simulink model "BuckyWagon_01"  (Simulink 7.7)
settings: Solver=FixedStepDiscrete  StartTime=0.0  StopTime=10.0  RelTol=1e-3
PreLoadFcn:
  | try, eval([bdroot '_setup']); catch, eval('model_setup', ''); end
InitFcn:
  | try, eval([bdroot '_setup']); catch, eval('model_setup', ''); end
undefined symbols (not defined in the file or in its folder): ECU565, High, Low, miniviewSetup, motohawk_build_version, motohawk_get_faults, motohawk_setup_toolchains, motohawk_trunc_name, motohawk_vardec_config_group, motohawk_vardec_path, tc, True
libraries: MotoHawk_lib x594, simulink x27, motohawk_control_primitives_lib x19, miniview_lib x10, MotoHawk_VDOGauge_lib x8, motohawk_engine_lib x5, motohawk_annotations_lib x1
(part 1 of 10)
Description:
  | ESled_08
CloseFcn:
  | try, eval([bdroot '_close']); catch, eval('model_close', ''); end
settings Model: MotoHawkBuildVersion=172  MotoHawkBuildStats=struct('TotalFLASH',{281540},'TotalEEPROM',{370},'TotalRAM',{18696},'AppFLASH',{71914},'AppEEPROM',{196},'AppRAM',{2166},'HeapRAM',{4096},'BuildSuccessCount',{175},'BuildErrorCount',{29},'OSRAM',{4754},'StackRAM',{7680},'FgndTimeStackSize',{3072},'FgndAngleStackSize',{0},'BgndStackSize',{2048},'IdleStackSize',{1024},'InterruptStackSize',{1536},'RTWBlockIOSize',{852},'RTWDWorkSize',{364},'RTWPrevZCSize',{0},'VolatileSize',{272},'NonVolatileSize',{196},'ConstantSize',{2208})  MotoHawkModelSavedName=BuckyWagon_01  MotoHawkModelGUID=3c32a120-d49a-4164-87-fe-ac-4b-55-ed-6f  MotoHawkModelOpenTime=2018 4 23 14 14 23.09  MotoHawkModelElapsedTime=-4921462.717  MotoHawkBuildInfo=struct('model_name',{'BuckyWagon_01'},'motohawk_version',{'2011a_sp0.184'},'motohawk_component_version',{'0.0.7'},'matlab_version',{'7.12.0'},'build_version',{'171'},'module_type',{'ECU565-128'},'layout_type',{'DEV'},'processor_family',{'PPC'},'processor_type',{'MPC565'},'toolchain_vendor',{'gcc-powerpc-eabi'},'toolchain_version',{'4.4.0'},'component',{0},'archive_file',{'PCM128.a'},'enable_build',{1},'fptype',{0},'flash_size',{1048576},'ee_size',{8192},'ram_size',{36864},'decram_size',{4096},'module_memory_def',{'MPC565_ModMemoryDef_Dev'},'eri_table0_rev',{9},'max_eri_table_size',{65535},'use_debug_vardecs',{1},'use_info_vardecs',{1},'fgnd_base_period_ms',{5},'bgnd_base_period_ms',{50},'root_build_dir',{'C:\Users\HYBRID\Documents\GitHub\Wisconsin-Hybrid\BuckyWagon_01'},'build_dir',{'C:\Users\HYBRID\Documents\GitHub\Wisconsin-Hybrid\BuckyWagon_01\BuckyWagon_01_Build'},'dll_name',{'BuckyWago_171'},'srz_name',{'BuckyWagon_01_171'},'fgnd_stack_size',{3072},'fgnd_angle_stack_size',{0},'bgnd_stack_size',{2048},'idle_stack_size',{1024},'irq_stack_size',{1536},'heap_size',{4096},'heap_margin',{409},'install_dll_dir',{'C:\ECUFiles\TDBDLL\'},'install_srz_dir',{'C:\ECUFiles\Programs'},'app_int_stack_size',{1024},'shutdown_stack_size',{1024},'mingw_dir',{'C:\PROGRA~2\Woodward\DEVELO~1\TOOLCH~1\GCC\win32-pe\4_4_0\'},'motohawk_dir',{'C:\PROGRA~2\Woodward\MCS\MotoHawk\2011A_~1.184'},'toolchain_dir',{'C:\Program Files (x86)\Woodward\DevelopmentTools\Toolchains\GCC\powerpc-eabi\4_4_0\'},'matlab_root',{'C:\Program Files (x86)\MATLAB\R2011a'},'model_guid',{'3c32a120-d49a-4164-87-fe-ac-4b-55-ed-6f'},'build_guid',{'f6bced0b-f3ce-4c1d-a0-1c-47-b3-99-ef-d3'},'token_guid',{'DD8AD11F95A6FC42BFF9AC780840E4B4'})  MotoHawkBuildGUID=f6bced0b-f3ce-4c1d-a0-1c-47-b3-99-ef-d3  Creator=Danny  LastModifiedBy=HYBRID
settings OptimizationCC: InlineParams=on  InitFltsAndDblsToZero=on  OptimizeModelRefInitCode=on  LifeSpan=1
settings DebuggingCC: SolverPrmCheckMsg=none  InheritedTsInSrcMsg=none  TasksWithSamePriorityMsg=none  StrictBusMsg=Warning
settings HardwareCC: ProdEndianess=BigEndian  ProdHWDeviceType=Specified
settings SFSimCC: SimCustomHeaderCode=|
  | #include <string.h>
  | #define charPtr(p) ((char *)p)
settings RTWCC: SystemTargetFile=motohawk_ert_rtw.tlc  TLCOptions="-aCustomNonFinites=\"motohawk_genrtnonfinite.tlc\""  MakeCommand=motohawk_make_rtw  TemplateMakefile=motohawk_ert_rtw.tmf  Description=MotoHawk(tm) Rapid Prototyping  ProcessScript=motohawk_ert_rtw_make_rtw_hook
settings CodeAppCC: IgnoreCustomStorageClasses=off  MaxIdLength=100  CustomSymbolStrField=$H$N$M
settings STFCustomTargetCC: FunctionExecutionProfile=off  ModelReferenceCompliant=off  CombineOutputUpdateFcns=on  ERTCustomFileBanners=on  SupportContinuousTime=off  SupportNonInlinedSFcns=off  SystemTargetFile=motohawk_ert_rtw.tlc
settings ERTTargetCC: FunctionExecutionProfile=off  MultiwordLength=2048  ModelReferenceCompliant=off  ParMdlRefBuildCompliant=off  CompOptLevelCompliant=off  ERTFirstTimeCompliant=off  ModelStepFunctionPrototypeControlCompliant=off  CPPClassGenCompliant=off  ERTCustomFileTemplate=example_file_process.tlc  ConvertIfToSwitch=off

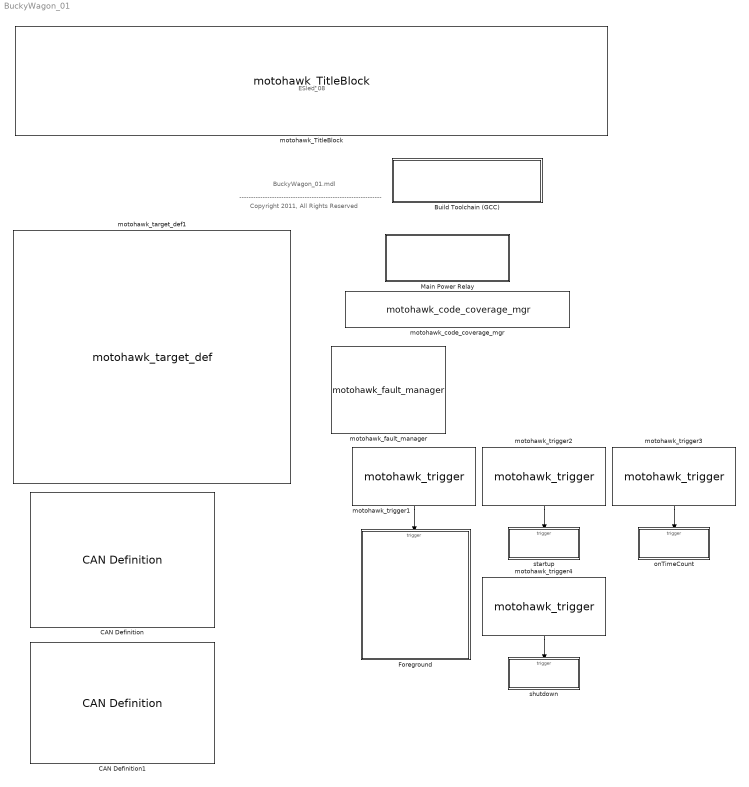
== system BuckyWagon_01 ==
  note: ESled_08
  note: BuckyWagon_01.mdl
  note: -------------------------------------------------------------
  note: Copyright 2011, All Rights Reserved
  Build Toolchain (GCC) : Subsystem
      mask Display:
      | patch([0 0 1 1], [0 1 1 0], [220/255 220/255 220/255]);
      | patch([0 0 1 1], [0 0.075 0.075 0], [230/255 0/255 0/255]);
      | patch([0 0 1 1], [0.025 0.05 0.05 0.025], [150/255 0/255 0/255]);
      | patch([0 0 1 1], [0 0.025 0.025 0], [0/255 0/255 0/255]);
      | 
      | disp(['Build'])
  CAN Definition : MotoHawk_lib/CAN Blocks/CAN Definition  Priority=-100  nam=['CAN_' num2str(1)]  text_resource=CAN1  code_resource=NONE  val_resource=-1  target=ECU565-128  bus=-2  btime=250 kbaud  pre=1  prop=0  pseg1=0  pseg2=0  resyn=0  tx_queue_size=16  rx_queue_size=16  use_protocol=on  city_id=hex2dec('B')  access_level=4  mototune_group='System | System Config | Communication Config'
  CAN Definition1 : MotoHawk_lib/CAN Blocks/CAN Definition  Priority=-100  nam=['CAN_' num2str(2)]  text_resource=CAN2  code_resource=NONE  val_resource=-1  target=ECU565-128  bus=-2  btime=500 kbaud  pre=1  prop=0  pseg1=0  pseg2=0  resyn=0  tx_queue_size=16  rx_queue_size=16  use_protocol=off  city_id=hex2dec('B')  access_level=4  mototune_group='System | System Config | Communication Config'
  Foreground : Subsystem  TreatAsAtomicUnit=on
      settings: RTWSystemCode=Function  RTWFcnNameOpts=Use subsystem name  RTWFileNameOpts=Use function name
  Main Power Relay : Subsystem  AncestorBlock=MotoHawk_lib/Extra Development Blocks/Main Power Relay  mask(MotoHawk Main Power Relay Control){on_delay_count=2, off_delay_count=10, ecup_threshold=100, group='System | Main Power Relay'}
      mask prompts: on_delay_count "On Delay Count"; off_delay_count "Off Delay Count"; ecup_threshold "ECUP High Threshold (ADC Counts)"; group "MotoTune Group"
      mask help:
      | This block provides basic control of the main power relay, by following the ECUP voltage input pin.
      |
      | Regardless of where the block is placed in a design, the strategy will execute every 50ms with background priority.
      |
      | Note that this block is simply composed of other primitive MotoHawk blocks and may be used as a starting point for a more complicated strategy.
      |
      | On Delay:  Once the ECU power goes high, after this period, the Main Power Relay will be turned on.
      | Off Delay:  Once the ECU power goes low, after this period, the Main Power Relay will be turned off.
      |
      | Note that one tick before MPRD is turned off, non-volatile variables will be stored, and the Shutdown event will be posted.  It is not necessary to use the Shutdown event.
      |
      | ---------------------------------------------------------------------
      |
      |
      | Copyright 2010 Woodward.  All Rights Reserved.
      mask init:
      | block = gcb;
      | 
      | motohawk_main_power_relay_initmask;
      mask Help: eval('motohawk_block_help(get_param(gcb,''MaskType''))');
      mask Display:
      | patch([0 0 1 1], [0 1 1 0], [220/255 220/255 220/255]);
      | patch([0 0 1 1], [0 0.075 0.075 0], [230/255 0/255 0/255]);
      | patch([0 0 1 1], [0.025 0.05 0.05 0.025], [150/255 0/255 0/255]);
      | patch([0 0 1 1], [0 0.025 0.025 0], [0/255 0/255 0/255]);
      | 
      | disp(['Main Power Relay' on_delay_lbl off_delay_lbl]);
  motohawk_TitleBlock : motohawk_annotations_lib/motohawk_TitleBlock  BlockType_='Mototron_Title_Block'  ttl="[  strrep(get_param(bdroot, 'Description') , '_', '\\_')  '\\newline\\rm'  'Top-level root of model:  '   strrep(bdroot, '_', '\\_') '.mdl'  ]"  copyright="'THE INFORMATION CONTAINED IN THIS\\newlineDRAWING IS THE SOLE PROPERTY OF\\newlineMOTOTRON.  ANY REPRODUCTION IN\\newline PART OR AS A WHOLE WITHOUT THE\\newlineWRITTEN PERMISSION OF MOTOTRON\\newline IS PROHIBITED.\\fontsize{16}\\rm\\copyright\\rm\\fontsize{10} 2005'"  address='\fontsize{22}\it\fontname{Arial Black}MotoTron Corporation \fontname{Arial}\fontsize{10}\newline505 Marion Road, Oshkosh, WI, 54901\newlinewww.mototron.com (734) 822-7700'  image_file='mh.jpg'  pretty_print=on  edit_text=|  edit_as=5
      | [	
      | 
      | 
      | 	
      | 
      | 
      | strrep(get_param(bdroot, 'Description') , '_', '\_')  '\newline\rm'	
      | 
      | 
      | 	
      | 
      | 
      | 'Top-level root of model:  '   strrep(bdroot, '_', '\_') '.mdl'	
      | 
      | 
      | 	
      | 
      | 
      | ]
  motohawk_code_coverage_mgr : MotoHawk_lib/Extra Development Blocks/motohawk_code_coverage_mgr  codegen=Always Generate Code Coverage Code  group='System | Code Coverage'
  motohawk_fault_manager : MotoHawk_lib/Fault Management Blocks/motohawk_fault_manager  storage=FLASH  read_level=1  write_level=1  clear_level=1  xytype=uint16  mototune_group='Faults'
  motohawk_target_def1 : MotoHawk_lib/motohawk_target_def  Priority=-65535  target=ECU565-128  layout=DEV  fptype=single (32 bits)  fgnd_stack_size=3*1024  fgnd_angle_stack_size=0  bgnd_stack_size=2*1024  idle_stack_size=1024  irq_stack_size=1536  app_int_stack_size=1024  shutdown_stack_size=1024  heap_size=4*1024  show_margins=off  fgnd_stack_margin=(3*1024) * 0.1  fgnd_angle_stack_margin=0  bgnd_stack_margin=(2*1024) * 0.1  idle_stack_margin=(1024) * 0.1  irq_stack_margin=(1536) * 0.1  app_int_stack_margin=(1024) * 0.1  shutdown_stack_margin=(1024) * 0.1  heap_margin=(4*1024) * 0.1  comp_name=bdroot  comp_img='KVASER_CAN_USB.jpg'  comp_security=No Encryption  comp_build_pass='mhbuild'  comp_sim_pass='mhsim'  comp_multi=off  show_filenames=off  dll_name=motohawk_trunc_name(bdroot, ['_' motohawk_build_version], 13)  srz_name=motohawk_trunc_name(bdroot, ['_' motohawk_build_version], 50)  build_dir='.'  comp_dir='.'
  motohawk_trigger1 : MotoHawk_lib/Trigger Blocks/motohawk_trigger  Tag=Trigger  trigger=FGND_RTI_PERIODIC  function_name=Trigger_FGND_RTI_PERIODIC_4287p0005  priority_order=0  inherited=off  run_disabled=off  override_app_monitor=off  target=ECU565_128
  motohawk_trigger2 : MotoHawk_lib/Trigger Blocks/motohawk_trigger  Tag=Trigger  trigger=STARTUP_EVENT  function_name=Trigger_STARTUP_EVENT_4288p0005  priority_order=0  inherited=off  run_disabled=off  override_app_monitor=off  target=ECU565_128
  motohawk_trigger3 : MotoHawk_lib/Trigger Blocks/motohawk_trigger  Tag=Trigger  trigger=BGND_BASEx20_PERIODIC  function_name=Trigger_BGND_BASEx20_PERIODIC_4289p0005  priority_order=0  inherited=off  run_disabled=off  override_app_monitor=off  target=ECU565_128
  motohawk_trigger4 : MotoHawk_lib/Trigger Blocks/motohawk_trigger  Tag=Trigger  Priority=0  trigger=SHUTDOWN_EVENT  function_name=Trigger_SHUTDOWN_EVENT_4290p0005  priority_order=0  inherited=off  run_disabled=off  override_app_monitor=off  target=ECU565_128
  onTimeCount : Subsystem  TreatAsAtomicUnit=on
  shutdown : Subsystem  TreatAsAtomicUnit=on
  startup : Subsystem  TreatAsAtomicUnit=on
  wires:
  motohawk_trigger1/1 -> Foreground/Trigger
  motohawk_trigger2/1 -> startup/Trigger
  motohawk_trigger3/1 -> onTimeCount/Trigger
  motohawk_trigger4/1 -> shutdown/Trigger

== system BuckyWagon_01/Build Toolchain (GCC) ==
  note: MotoHawk
  note: ---------------------------------------------------------------------
      | Copyright 2010 Woodward.  All Rights Reserved.
  note: Build Blocks
  Tool Chain Definition : S-Function  InitFcn=motohawk_setup_toolchains(gcb, 'init');  FunctionName=motohawk_sfun_toolchain_def  Parameters=char({tc,''})  EnableBusSupport=off  mask(MotoHawk Tool Chain Definition){nam='MyToolChain', toolchain=gcc-powerpc-eabi 4.4.0, buildtemplate=GreenHills 3.6, toolchaindir='C:\\GHS\\ppc421\\', target=ECU565-128}
      mask prompts: nam "Name"; toolchain "Tool Chain"; buildtemplate "Build Template"; toolchaindir "Tool Chain Install Directory"; target "Target (hidden)"
      mask help:
      | This block chooses the tool chain for MotoHawk to use when CTRL+B is pressed.
      |
      | The "Name" is a user-specified name given to the tool chain.  It has no bearing on the tool chain chosen, it is for documentation purposes.
      |
      | The "Tool Chain" drop down list contains the tool chains that are available for this target.
      |
      | A "Custom" toolchain allows the user to choose an alternate directory with a supported build template.
      |
      | The "Build template" will force MotoHawk to generate build scripts and files for the specified tool chain.  Note that a custom tool chain must be compatible with a supported tool chain, otherwise the build will not succeed.
      |
      | ---------------------------------------------------------------------
      |
      |
      | Copyright 2010 Woodward.  All Rights Reserved.
      mask init:
      | block = gcb;
      | 
      | motohawk_sfun_toolchain_def_initmask;
      settings: OpenFcn=|
      | motohawk_setup_toolchains(gcb, 'open');
      | open_system(gcb, 'mask');
      mask Help: eval('motohawk_block_help(get_param(gcb,''MaskType''))');
      mask StyleString: edit,popup((None)|(Custom)|GreenHills 3.6|GreenHills 4.2.1|gcc-powerpc-eabi 4.4.0),popup(GreenHills 3.6|GreenHills 4.2.1|gcc-powerpc-eabi 4.4.0),edit,edit
      mask CallbackString: |motohawk_sfun_toolchain_def_visible(gcb)|||
      mask Display:
      | patch([0 0 1 1], [0 1 1 0], [220/255 220/255 220/255]);
      | 
      | patch([0 0 1 1], [0 0.075 0.075 0], [230/255 0/255 0/255]);
      | patch([0 0 1 1], [0.025 0.05 0.05 0.025], [150/255 0/255 0/255]);
      | 
      | patch([0 0 1 1], [0 0.025 0.025 0], [0/255 0/255 0/255]);
      | 
      | 
      | text(0.1, 0.9, lbl, 'texmode', 'on', 'HorizontalAlignment', 'Left', 'VerticalAlignment', 'Top');

== system BuckyWagon_01/Foreground ==
  function : TriggerPort  TriggerType=function-call
  Actuators : Subsystem
  Addl_Fault_Detection : Subsystem
  Control Strategy : Subsystem
  Gauges : Subsystem
  MiniViewDisplay : Subsystem
      settings: RTWSystemCode=Function  RTWFcnNameOpts=Use subsystem name  RTWFileNameOpts=Use function name
  Sensors : Subsystem
  motohawk_trigger : MotoHawk_lib/Trigger Blocks/motohawk_trigger  Tag=Trigger  trigger=FGND_RTI_PERIODIC  function_name=Trigger_FGND_RTI_PERIODIC_4085p0005  priority_order=200  inherited=on  run_disabled=off  override_app_monitor=off  target=ECU565_128
  motohawk_trigger1 : MotoHawk_lib/Trigger Blocks/motohawk_trigger  Tag=Trigger  trigger=FGND_20XRTI_PERIODIC  function_name=Trigger_FGND_20XRTI_PERIODIC_4086p0002  priority_order=200  inherited=on  run_disabled=off  override_app_monitor=off  target=ECU565_128
  wires:
  Sensors/1(Sensors) -> Control Strategy/1(Inputs), Gauges/1(Inputs), MiniViewDisplay/1(Inputs), Addl_Fault_Detection/1(In1)  "Physical"
  Control Strategy/1(Outputs) -> Actuators/1(Outputs), MiniViewDisplay/2(Outputs), Gauges/2(Outputs)  "Hybrid"
  motohawk_trigger/1 -> MiniViewDisplay/Trigger
  motohawk_trigger1/1 -> Gauges/Trigger

== system BuckyWagon_01/Main Power Relay ==
  note: Always execute Main Power Relay control in the background.
  note: The saving and restoring of non-volatile variables
      | must be called from a background priority task.
  Background : Subsystem
  motohawk_trigger : MotoHawk_lib/Trigger Blocks/motohawk_trigger  Tag=Trigger  Priority=255  trigger=BGND_BASE_PERIODIC  function_name=Trigger_BGND_BASE_PERIODIC_4279p0005  priority_order=255  inherited=on  run_disabled=on  override_app_monitor=off  target=ECU565_128
  wires:
  motohawk_trigger/1 -> Background/Trigger

== system BuckyWagon_01/onTimeCount ==
  function : TriggerPort  TriggerType=function-call
  Constant : Constant  OutDataTypeStr=uint32
  Sum : Sum  Inputs=++|
  motohawk_data_def : MotoHawk_lib/Data Storage Blocks/motohawk_data_def  nam='totalOnTime'  container_nam=''  data=0  typ=uint32  struct_nam='MyStruct'  storage=NonVolatile  outputRef=on  use_vardec=on  window=Display  read_level=1  write_level=1  ovr_cals=on  view_as=Number  enum_struct={'Disabled', 'Enabled'}  vector_style=Wide Row  use_help_units=off  help=''  units=''  use_header_enum=off  row_header_enum=''  col_header_enum=''  use_min_max=off  min_val=-inf  max_val=inf  use_precision=off  precision=''  gain=1  offset=0  exp=1  use_mototune_group=off  mototune_group=motohawk_vardec_path(gcb)  eval_name=MyData  data_stores=motohawk_sfun_data_def_data_stores  struct_instances=motohawk_sfun_data_def_struct_instances  vardecs=motohawk_sfun_data_def_vardecs
  motohawk_data_read : MotoHawk_lib/Data Storage Blocks/motohawk_data_read  source=Input Reference Signal  structure=Scalar  operation=Read scalar from location by index  sz_vec=4  sz_row=2  sz_col=3  typ=uint32  nam='MyData'  checkNull=on  struct_inst_name=''  struct_nam='MyStruct'
  motohawk_data_write : MotoHawk_lib/Data Storage Blocks/motohawk_data_write  source=Input Reference Signal  structure=Scalar  operation=Write entire data structure at once  sz_vec=9  sz_row=2  sz_col=9  typ=uint32  nam='MyData'  checkNull=on  write_read_only=off  struct_inst_name=''  struct_name='MyStruct'
  wires:
  Constant/1 -> Sum/1
  Sum/1 -> motohawk_data_write/1
  motohawk_data_read/1 -> Sum/2
  motohawk_data_def/1 -> motohawk_data_write/2, motohawk_data_read/1

== system BuckyWagon_01/shutdown ==
  note: Note: this does not currently do anything, See startup (that does the things)
  function : TriggerPort  TriggerType=function-call
  VDO Gauge Reset : MotoHawk_VDOGauge_lib/VDO Gauge Reset  nam='GaugeChain'

== system BuckyWagon_01/startup ==
  function : TriggerPort  TriggerType=function-call
  Constant : Constant  OutDataTypeStr=uint32
  Sum : Sum  Inputs=++|
  VDO Gauge Reset : MotoHawk_VDOGauge_lib/VDO Gauge Reset  nam='GaugeChain'
  motohawk_data_def : MotoHawk_lib/Data Storage Blocks/motohawk_data_def  nam='startupCount'  container_nam=''  data=0  typ=uint32  struct_nam='MyStruct'  storage=NonVolatile  outputRef=on  use_vardec=on  window=Display  read_level=1  write_level=1  ovr_cals=on  view_as=Number  enum_struct={'Disabled', 'Enabled'}  vector_style=Wide Row  use_help_units=off  help=''  units=''  use_header_enum=off  row_header_enum=''  col_header_enum=''  use_min_max=off  min_val=-inf  max_val=inf  use_precision=off  precision=''  gain=1  offset=0  exp=1  use_mototune_group=off  mototune_group=motohawk_vardec_path(gcb)  eval_name=MyData  data_stores=motohawk_sfun_data_def_data_stores  struct_instances=motohawk_sfun_data_def_struct_instances  vardecs=motohawk_sfun_data_def_vardecs
  motohawk_data_read : MotoHawk_lib/Data Storage Blocks/motohawk_data_read  source=Input Reference Signal  structure=Scalar  operation=Read scalar from location by index  sz_vec=4  sz_row=2  sz_col=3  typ=uint32  nam='MyData'  checkNull=on  struct_inst_name=''  struct_nam='MyStruct'
  motohawk_data_write : MotoHawk_lib/Data Storage Blocks/motohawk_data_write  source=Input Reference Signal  structure=Scalar  operation=Write entire data structure at once  sz_vec=9  sz_row=2  sz_col=9  typ=uint32  nam='MyData'  checkNull=on  write_read_only=off  struct_inst_name=''  struct_name='MyStruct'
  wires:
  motohawk_data_def/1 -> motohawk_data_read/1, motohawk_data_write/2
  motohawk_data_read/1 -> Sum/2
  Sum/1 -> motohawk_data_write/1
  Constant/1 -> Sum/1

== system BuckyWagon_01/Foreground/Actuators ==
  note: Delete this eventually
      | A.K.A next major code flash
  Outputs : Inport
  A123 Battery Controller : Subsystem  TreatAsAtomicUnit=on
  Analog Out : Subsystem  TreatAsAtomicUnit=on
  Brusa Charger : Subsystem  AncestorBlock=motohawk_annotations_lib/Display Image File  mask(Display Image File){image_file='NLG5.jpg'}
      mask prompts: image_file "Image File"
      mask help:
      | Enter an image file on the current MATLAB path to display on this block.
      |
      | Double-clicking this block opens the contents of the subsystem.  Right-click and select 'Mask parameters...' to select a new image file.
      |
      | To use just the mask of this block in a model, but supply your own contents, break the link to the library.
      mask init:
      | try,
      | 	img = imread(image_file);
      | 	motohawk_block_image(gcb, image_file);
      | catch,
      | 	img = imread('image_not_found.jpg');
      | end
      settings: OpenFcn=open_system(gcb,'force');  MoveFcn=motohawk_block_image(gcb, motohawk_get_param_ws(gcb, 'image_file'));
      mask Display: image(img);
  Bus Selector1 : BusSelector  OutputSignals=Drive Enable,Motor_Torque
  Bus Selector2 : BusSelector  OutputSignals=InReverse,FanDutyCycle,DC/DC Enable,Brake
  Bus Selector3 : BusSelector  OutputSignals=Contactor Command
  Bus Selector4 : BusSelector  OutputSignals=EHPAS_enable
  Bus Selector5 : BusSelector  OutputSignals=NLG5
  Bus Selector6 : BusSelector  OutputSignals=Motor_Torque
  Bus Selector8 : BusSelector  OutputSignals=CoolantPumpSpeed
  EHPAS Power Steering Pump Controller : Subsystem  TreatAsAtomicUnit=on
  EMP Coolant Pump : Subsystem  TreatAsAtomicUnit=on
  Eaton Controller : Subsystem
  Eaton HV Charger : Subsystem  AncestorBlock=motohawk_annotations_lib/Display Image File  mask(Display Image File){image_file='NLG5.jpg'}
      mask prompts: image_file "Image File"
      mask help:
      | Enter an image file on the current MATLAB path to display on this block.
      |
      | Double-clicking this block opens the contents of the subsystem.  Right-click and select 'Mask parameters...' to select a new image file.
      |
      | To use just the mask of this block in a model, but supply your own contents, break the link to the library.
      mask init:
      | try,
      | 	img = imread(image_file);
      | 	motohawk_block_image(gcb, image_file);
      | catch,
      | 	img = imread('image_not_found.jpg');
      | end
      settings: OpenFcn=open_system(gcb,'force');  MoveFcn=motohawk_block_image(gcb, motohawk_get_param_ws(gcb, 'image_file'));
  Solectria Controller : Subsystem
  Terminator : Terminator
  motohawk_calibration2 : MotoHawk_lib/Calibration & Probing Blocks/motohawk_calibration  nam='Enable_PowerSteering_CAN_Msg'  val=1  storage=Calibration  show_more=on  name_source=Use Parameter  data_type=boolean  read_level=1  write_level=1  ovr_cals=on  view_as=Number  enum_struct={'Disabled', 'Enabled'}  vector_style=Wide Row  use_help_units=off  help=''  units=''  use_header_enum=off  row_header_enum={}  col_header_enum={}  use_min_max=off  min_val=-inf  max_val=inf  use_precision=on  precision=''  gain=1  offset=0  exp=1  use_mototune_group=off  mototune_group=motohawk_vardec_path(gcb)
  wires:
  Outputs/1 -> Bus Selector3/1, Bus Selector1/1, Bus Selector4/1, Bus Selector5/1, Bus Selector2/1, Bus Selector8/1, Eaton HV Charger/1(In), Eaton Controller/2(Inputs), Bus Selector6/1
  Bus Selector8/1 -> EMP Coolant Pump/1(PercentSpeed)  "<CoolantPumpSpeed>"
  Bus Selector5/1 -> Brusa Charger/1(In1)  "<NLG5>"
  Bus Selector1/2 -> Solectria Controller/1(Motor Torque), Eaton Controller/1(Motor Torque)  "<Motor_Torque>"
  Bus Selector3/1 -> A123 Battery Controller/1(Contactor Command)  "<Contactor Command>"
  Bus Selector1/1 -> Terminator/1  "<Drive Enable>"
  Bus Selector4/1 -> EHPAS Power Steering Pump Controller/1(Enable)  "<EHPAS_enable>"
  [PluggedIn] -> Brusa Charger/Enable
  Bus Selector2/1 -> Analog Out/1(In Reverse)  "<InReverse>"
  Bus Selector2/2 -> Analog Out/2(Fan Duty Cycle)  "<FanDutyCycle>"
  Bus Selector2/3 -> Analog Out/3(Enable)  "<DC/DC Enable>"
  Bus Selector2/4 -> Analog Out/4(Brake)  "<Brake>"
  motohawk_calibration2/1 -> EHPAS Power Steering Pump Controller/Enable
  Bus Selector6/1 -> A123 Battery Controller/2(Torque Request)  "<Motor_Torque>"

== system BuckyWagon_01/Foreground/Addl_Fault_Detection ==
  In1 : Inport
  Battery : Subsystem
  Bus Selector1 : BusSelector  OutputSignals=LVVoltage
  Bus Selector2 : BusSelector  OutputSignals=SOC,DC_Voltage,MCUDCVoltage,ContactorStatus
  Bus Selector3 : BusSelector  OutputSignals=LVVoltage,VehicleSpeed,MotorTorque,Accel
  LowVoltageSystem : Subsystem
  Traction Drive : Subsystem
  wires:
  In1/1 -> Bus Selector2/1, Bus Selector1/1, Bus Selector3/1  "Inputs"
  Bus Selector1/1 -> LowVoltageSystem/1(12V system Voltage)  "<LVVoltage>"
  Bus Selector2/1 -> Battery/1(SOC)  "<SOC>"
  Bus Selector2/2 -> Battery/2(Battery Voltage)  "<DC_Voltage>"
  Bus Selector2/3 -> Battery/3(Motor/ steering voltage)  "<MCUDCVoltage>"
  Bus Selector2/4 -> Battery/4(Contactor status)  "<ContactorStatus>"
  Bus Selector3/1 -> Traction Drive/1(Accel)  "<LVVoltage>"
  Bus Selector3/2 -> Traction Drive/2(Vehcile Speed)  "<VehicleSpeed>"
  Bus Selector3/3 -> Traction Drive/3(Motor Torque)  "<MotorTorque>"
  Bus Selector3/4 -> Traction Drive/4(Accel1)  "<Accel>"

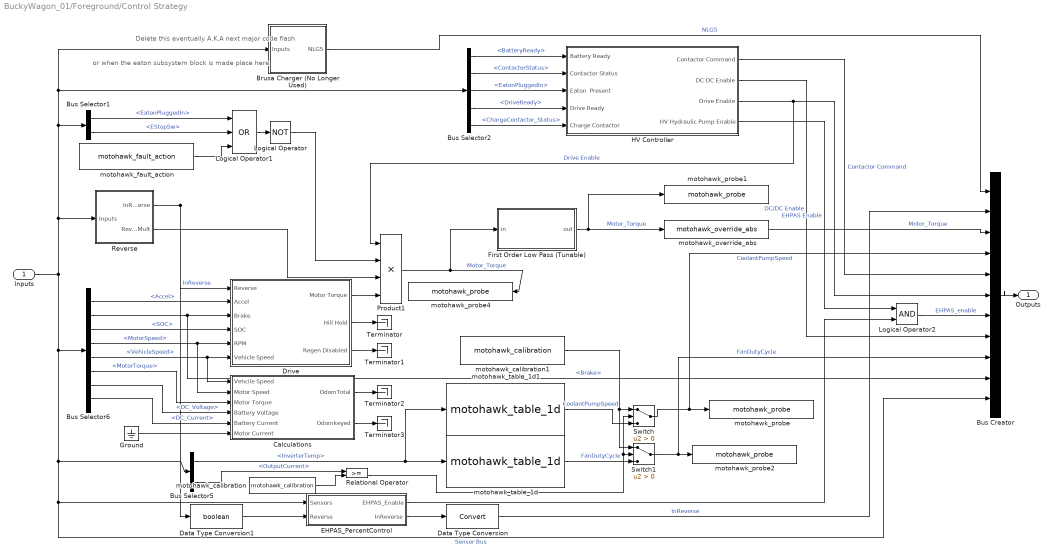
== system BuckyWagon_01/Foreground/Control Strategy ==
  note: Delete this eventually
      | A.K.A next major code flash
  note: or when the eaton subsystem block is made place here
  Inputs : Inport
  Brusa Charger (No Longer Used) : Subsystem  TreatAsAtomicUnit=on
  Bus Creator : BusCreator  Inputs=11
  Bus Selector1 : BusSelector  OutputSignals=Eaton HV Charger.EatonPluggedIn,EStopSw
  Bus Selector2 : BusSelector  OutputSignals=BatteryReady,ContactorStatus,Eaton HV Charger.EatonPluggedIn,DriveReady,ChargeContactor_Status
  Bus Selector5 : BusSelector  OutputSignals=InverterTemp,Eaton HV Charger.OutputCurrent
  Bus Selector6 : BusSelector  OutputSignals=Accel,Brake,SOC,MotorSpeed,VehicleSpeed,MotorTorque,DC_Voltage,DC_Current
  Calculations : Subsystem
  Data Type Conversion : DataTypeConversion
  Data Type Conversion1 : DataTypeConversion  OutDataTypeStr=boolean
  Drive : Subsystem  TreatAsAtomicUnit=on
  EHPAS_PercentControl : Subsystem
  First Order Low Pass (Tunable) : Subsystem  mask(First-Order Low-Pass Filter (Tunable)){nam='FiltConst', samp_time=-1, group=motohawk_vardec_path(gcb)}
      mask prompts: nam "Name"; samp_time "Sample Time"; group "MotoTune Group String"
      mask help:
      | Discrete first-order low-pass filter, with calibratable time-constant.
      |
      | If 'Sample Time' is -1, then extra code and RAM will be generated to dynamically calculate dt.
      mask Display:
      | patch([0 0 1 1], [0 0.075 0.075 0], [230/255 0/255 0/255])
      | patch([0 0 1 1], [0.025 0.05 0.05 0.025], [150/255 0/255 0/255])
      | patch([0 0 1 1], [0 0.025 0.025 0], [0/255 0/255 0/255])
      | 
      | disp('1st-Order\nLow Pass');
  Ground : Ground
  HV Controller : Subsystem  TreatAsAtomicUnit=on
  Logical Operator : Logic  Operator=NOT  AllPortsSameDT=off  OutDataTypeStr=boolean
  Logical Operator1 : Logic  Operator=OR  Inputs=3  AllPortsSameDT=off  OutDataTypeStr=boolean
  Logical Operator2 : Logic  AllPortsSameDT=off  OutDataTypeStr=boolean
  Product1 : Product  Inputs=4  RndMeth=Zero
  Relational Operator : RelationalOperator  OutDataTypeStr=boolean
  Reverse : Subsystem  TreatAsAtomicUnit=on
  Switch : Switch  Criteria=u2 > Threshold
  Switch1 : Switch  Criteria=u2 > Threshold
  Terminator{,1..3} (4 alike) : Terminator
  motohawk_calibration : MotoHawk_lib/Calibration & Probing Blocks/motohawk_calibration  nam='Charger_Curr'  val=8  storage=Calibration  show_more=off  name_source=Use Parameter  data_type=Inherit from 'Default Value'  read_level=1  write_level=1  ovr_cals=on  view_as=Number  enum_struct={'Disabled', 'Enabled'}  vector_style=Wide Row  use_help_units=off  help=''  units=''  use_header_enum=off  row_header_enum={}  col_header_enum={}  use_min_max=off  min_val=-inf  max_val=inf  use_precision=off  precision=''  gain=1  offset=0  exp=1  use_mototune_group=off  mototune_group=motohawk_vardec_path(gcb)
  motohawk_calibration1 : MotoHawk_lib/Calibration & Probing Blocks/motohawk_calibration  nam='Charging_Cooling_Speed'  val=40  storage=Calibration  show_more=off  name_source=Use Parameter  data_type=Inherit from 'Default Value'  read_level=1  write_level=1  ovr_cals=on  view_as=Number  enum_struct={'Disabled', 'Enabled'}  vector_style=Wide Row  use_help_units=off  help=''  units=''  use_header_enum=off  row_header_enum={}  col_header_enum={}  use_min_max=off  min_val=-inf  max_val=inf  use_precision=off  precision=''  gain=1  offset=0  exp=1  use_mototune_group=off  mototune_group=motohawk_vardec_path(gcb)
  motohawk_fault_action : MotoHawk_lib/Fault Management Blocks/motohawk_fault_action  nam='DisableDrive'  output_status=on  eval_nam=DisableDrive
  motohawk_override_abs : MotoHawk_lib/Calibration & Probing Blocks/motohawk_override_abs  SystemSampleTime=-1  parent_name='motor_torque_Ovr'  parent_val=0  show_more=off  name_source=Use Parameter  parent_read_level=1  parent_override_level=1  view_as=Number  enum_struct={'Disabled', 'Enabled'}  use_help_units=off  parent_help=''  parent_units=''  use_min_max=off  parent_min=-inf  parent_max=inf  use_precision=off  parent_precision=''  parent_gain=1  parent_offset=0  parent_exp=1  use_mototune_group=off  parent_group=motohawk_vardec_path(gcb)
  motohawk_probe : MotoHawk_lib/Calibration & Probing Blocks/motohawk_probe  nam='CoolantPumpSpeed_out'  show_more=off  name_source=Use Parameter  read_level=1  view_as=Number  enum_struct={'Disabled', 'Enabled'}  vector_style=Wide Row  use_help_units=off  help=''  units=''  use_header_enum=off  row_header_enum={}  col_header_enum={}  use_precision=off  precision=''  gain=1  offset=0  exp=1  use_mototune_group=off  mototune_group=motohawk_vardec_path(gcb)
  motohawk_probe1 : MotoHawk_lib/Calibration & Probing Blocks/motohawk_probe  nam='motor_Torque'  show_more=on  name_source=Use Parameter  read_level=1  view_as=Number  enum_struct={'Disabled', 'Enabled'}  vector_style=Wide Row  use_help_units=off  help=''  units=''  use_header_enum=off  row_header_enum={}  col_header_enum={}  use_precision=on  precision='1.3'  gain=1  offset=0  exp=1  use_mototune_group=off  mototune_group=motohawk_vardec_path(gcb)
  motohawk_probe2 : MotoHawk_lib/Calibration & Probing Blocks/motohawk_probe  nam='RadiatorFanSpeed_out'  show_more=off  name_source=Use Parameter  read_level=1  view_as=Number  enum_struct={'Disabled', 'Enabled'}  vector_style=Wide Row  use_help_units=off  help=''  units=''  use_header_enum=off  row_header_enum={}  col_header_enum={}  use_precision=off  precision=''  gain=1  offset=0  exp=1  use_mototune_group=off  mototune_group=motohawk_vardec_path(gcb)
  motohawk_probe4 : MotoHawk_lib/Calibration & Probing Blocks/motohawk_probe  nam='pre_Filter_Torque_Request'  show_more=off  name_source=Use Parameter  read_level=1  view_as=Number  enum_struct={'Disabled', 'Enabled'}  vector_style=Wide Row  use_help_units=off  help=''  units=''  use_header_enum=off  row_header_enum={}  col_header_enum={}  use_precision=off  precision=''  gain=1  offset=0  exp=1  use_mototune_group=off  mototune_group=motohawk_vardec_path(gcb)
  motohawk_table_1d : MotoHawk_lib/Lookup Tables/motohawk_table_1d  SystemSampleTime=-1  nam='RadiatorFanSpeed'  bp_nam='RadiatorFanSpeed_InverterTemp'  breakpoint_data=[0 20 30 45 100]  table_data=[0 0 0 30 50]  show_more=off  bp_data_type=Inherit from 'Breakpoint Data'  bp_storage=Constant  table_data_type=Inherit from 'Table Data'  storage=NonAdaptive  read_level=1  write_level=1  ovr_cals=on  use_help=off  help=''  bp_units=''  table_units=''  use_min_max=off  bp_min_val=-inf  bp_max_val=inf  min_val=-inf  max_val=inf  use_precision=off  use_breakpoint=off  b_precision=''  b_gain=1  b_offset=0  b_exp=1  use_table=off  t_precision=''  t_gain=1  t_offset=0  t_exp=1  use_links=off  input_name=''  output_name=''  use_mototune_group=off  mototune_group=motohawk_vardec_path(gcb)
  motohawk_table_1d1 : MotoHawk_lib/Lookup Tables/motohawk_table_1d  SystemSampleTime=-1  nam='CoolantPumpSpeed'  bp_nam=''  breakpoint_data=[0 10 28 30 35 40 60 70 80 90 100]  table_data=[20 25 35 45 53 65 75 80 80 80 80]  show_more=on  bp_data_type=Inherit from 'Breakpoint Data'  bp_storage=Constant  table_data_type=Inherit from 'Table Data'  storage=NonAdaptive  read_level=1  write_level=1  ovr_cals=on  use_help=off  help=''  bp_units=''  table_units=''  use_min_max=off  bp_min_val=-inf  bp_max_val=inf  min_val=-inf  max_val=inf  use_precision=off  use_breakpoint=off  b_precision=''  b_gain=1  b_offset=0  b_exp=1  use_table=off  t_precision=''  t_gain=1  t_offset=0  t_exp=1  use_links=off  input_name=''  output_name=''  use_mototune_group=off  mototune_group=motohawk_vardec_path(gcb)
  Outputs : Outport
  wires:
  Inputs/1 -> Reverse/1(Inputs), Bus Selector1/1, Bus Selector2/1, Brusa Charger (No Longer Used)/1(Inputs), Bus Selector6/1, Bus Selector5/1, EHPAS_PercentControl/1(Sensors), Bus Creator/11  "Sensor Bus"
  Reverse/2(ReverseMult) -> Product1/3
  Logical Operator/1 -> Product1/2
  Bus Creator/1 -> Outputs/1
  motohawk_fault_action/1 -> Logical Operator1/3
  Logical Operator1/1 -> Logical Operator/1
  Brusa Charger (No Longer Used)/1(NLG5) -> Bus Creator/1  "NLG5"
  Bus Selector2/1 -> HV Controller/1(Battery Ready)  "<BatteryReady>"
  Bus Selector2/2 -> HV Controller/2(Contactor Status)  "<ContactorStatus>"
  HV Controller/1(Contactor Command) -> Bus Creator/5  "Contactor Command"
  HV Controller/3(Drive Enable) -> Bus Creator/6, Product1/1  "Drive Enable"
  HV Controller/2(DC DC Enable) -> Bus Creator/8  "DC/DC Enable"
  Bus Selector2/3 -> HV Controller/3(Eaton  Present)  "<EatonPluggedIn>"
  Drive/1(Motor Torque) -> Product1/4
  Product1/1 -> First Order Low Pass (Tunable)/1(in), motohawk_probe4/1  "Motor_Torque"
  Bus Selector6/1 -> Drive/2(Accel)  "<Accel>"
  Bus Selector6/2 -> Drive/3(Brake), Bus Creator/10  "<Brake>"
  Bus Selector6/3 -> Drive/4(SOC)  "<SOC>"
  Bus Selector6/4 -> Drive/5(RPM), Calculations/2(Motor Speed)  "<MotorSpeed>"
  Bus Selector6/5 -> Calculations/1(Vehcile Speed), Drive/6(Vehicle Speed)  "<VehicleSpeed>"
  Bus Selector6/6 -> Calculations/3(Motor Torque)  "<MotorTorque>"
  Bus Selector6/7 -> Calculations/4(Battery Voltage)  "<DC_Voltage>"
  Bus Selector6/8 -> Calculations/5(Battery Current)  "<DC_Current>"
  Bus Selector1/1 -> Logical Operator1/1  "<EatonPluggedIn>"
  Bus Selector5/1 -> motohawk_table_1d/1, motohawk_table_1d1/1  "<InverterTemp>"
  Bus Selector1/2 -> Logical Operator1/2  "<EStopSw>"
  Drive/2(Hill Hold) -> Terminator/1
  Drive/3(Regen Disabled) -> Terminator1/1
  Calculations/1(OdomTotal) -> Terminator2/1
  Calculations/2(Odomkeyed) -> Terminator3/1
  Ground/1 -> Calculations/6(Motor Current)
  Bus Selector2/4 -> HV Controller/4(Drive Ready)  "<DriveReady>"
  Bus Selector2/5 -> HV Controller/5(Charge Contactor)  "<ChargeContactor_Status>"
  First Order Low Pass (Tunable)/1(out) -> motohawk_probe1/1, motohawk_override_abs/1  "Motor_Torque"
  Logical Operator2/1 -> Bus Creator/7  "EHPAS_enable"
  HV Controller/4(HV Hydraulic Pump Enable) -> Logical Operator2/1  "EHPAS Enable"
  EHPAS_PercentControl/1(EHPAS_Enable) -> Logical Operator2/2
  EHPAS_PercentControl/2(InReverse) -> Data Type Conversion/1
  Data Type Conversion/1 -> Bus Creator/2  "InReverse"
  Data Type Conversion1/1 -> EHPAS_PercentControl/2(Reverse)
  Reverse/1(InReverse) -> Data Type Conversion1/1, Drive/1(Reverse)  "InReverse"
  motohawk_override_abs/1 -> Bus Creator/3  "Motor_Torque"
  Bus Selector5/2 -> Relational Operator/1  "<OutputCurrent>"
  motohawk_calibration/1 -> Relational Operator/2
  motohawk_table_1d1/1 -> Switch/3  "CoolantPumpSpeed"
  motohawk_table_1d/1 -> Switch1/3  "FanDutyCycle"
  Switch1/1 -> motohawk_probe2/1, Bus Creator/9  "FanDutyCycle"
  Switch/1 -> motohawk_probe/1, Bus Creator/4  "CoolantPumpSpeed"
  Relational Operator/1 -> Switch1/2, Switch/2
  motohawk_calibration1/1 -> Switch/1, Switch1/1

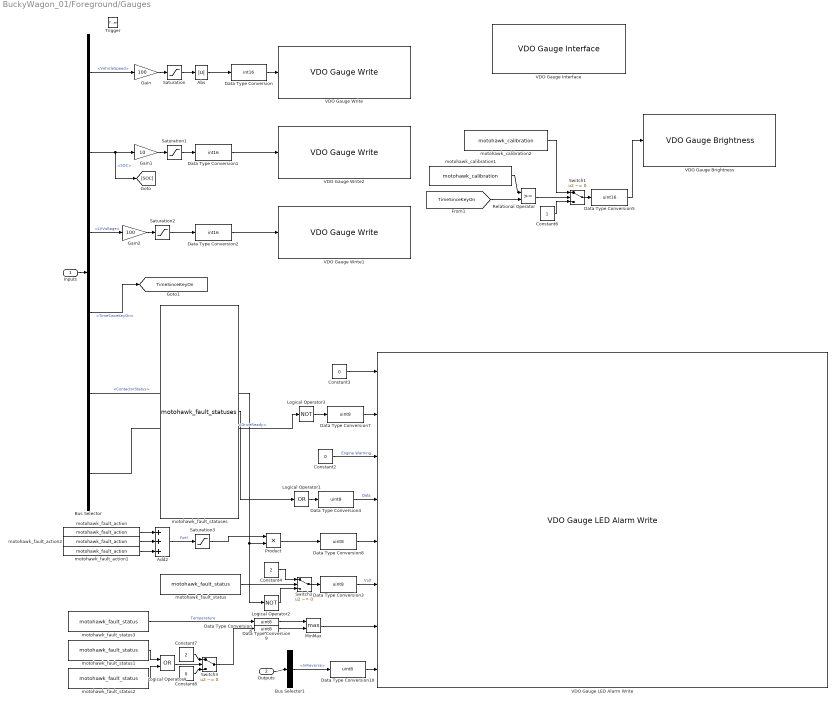
== system BuckyWagon_01/Foreground/Gauges ==
  Inputs : Inport
  Outputs : Inport  Port=2
  Trigger : TriggerPort  TriggerType=function-call
  Abs : Abs
  Add2 : Sum  Inputs=+++  AccumDataTypeStr=uint8
  Bus Selector : BusSelector  OutputSignals=VehicleSpeed,SOC,LVVoltage,TimeSinceKeyOn,ContactorStatus,DriveReady
  Bus Selector1 : BusSelector  OutputSignals=InReverse
  Constant2 : Constant  Value=0  OutDataTypeStr=uint8
  Constant3 : Constant  Value=0  OutDataTypeStr=uint8
  Constant4 : Constant  Value=2  OutDataTypeStr=uint8
  Constant6 : Constant  OutDataTypeStr=int16
  Constant7 : Constant  Value=2  OutDataTypeStr=uint8
  Constant8 : Constant  Value=0  OutDataTypeStr=uint8
  Data Type Conversion : DataTypeConversion  OutDataTypeStr=int16
  Data Type Conversion1 : DataTypeConversion  OutDataTypeStr=int16
  Data Type Conversion{3..4,6..10} (7 alike) : DataTypeConversion  OutDataTypeStr=uint8
  Data Type Conversion2 : DataTypeConversion  OutDataTypeStr=int16
  Data Type Conversion5 : DataTypeConversion  OutDataTypeStr=uint16
  Gain : Gain  Gain=100
  Gain1 : Gain  Gain=10
  Gain2 : Gain  Gain=100
  Logical Operator1 : Logic  Operator=OR  Inputs=1  AllPortsSameDT=off  OutDataTypeStr=boolean
  Logical Operator2 : Logic  Operator=NOT  Inputs=1  AllPortsSameDT=off  OutDataTypeStr=boolean
  Logical Operator3 : Logic  Operator=NOT  Inputs=1  AllPortsSameDT=off  OutDataTypeStr=boolean
  Logical Operator4 : Logic  Operator=OR  AllPortsSameDT=off  OutDataTypeStr=boolean
  MinMax : MinMax  Function=max  Inputs=2
  Product : Product  RndMeth=Zero
  Relational Operator : RelationalOperator  OutDataTypeStr=boolean
  Saturation : Saturate  UpperLimit=+10000  LowerLimit=-10000
  Saturation1 : Saturate  UpperLimit=1000  LowerLimit=0
  Saturation2 : Saturate  UpperLimit=2000  LowerLimit=0
  Saturation3 : Saturate  UpperLimit=2  LowerLimit=0
  Switch1 : Switch  Criteria=u2 ~= 0
  Switch2 : Switch  Criteria=u2 ~= 0
  Switch3 : Switch  Criteria=u2 ~= 0
  VDO Gauge Brightness : MotoHawk_VDOGauge_lib/VDO Gauge Brightness  nam='GaugeChain'  per=2000
  VDO Gauge Interface : MotoHawk_VDOGauge_lib/VDO Gauge Interface  nam='GaugeChain'  text_resource=TACH  code_resource=NONE  val_resource=-1  target=ECU565-128  dly=1600  queue_size=128  dyn_create=off
  VDO Gauge LED Alarm Write : MotoHawk_VDOGauge_lib/VDO Gauge LED Alarm Write  nam='GaugeChain'  pri=(None)
  VDO Gauge Write : MotoHawk_VDOGauge_lib/VDO Gauge Write  nam='GaugeChain'  res=Speed  pri=(None)
  VDO Gauge Write1 : MotoHawk_VDOGauge_lib/VDO Gauge Write  nam='GaugeChain'  res=Voltage  pri=(None)
  VDO Gauge Write2 : MotoHawk_VDOGauge_lib/VDO Gauge Write  nam='GaugeChain'  res=Fuel Level  pri=(None)
  motohawk_calibration1 : MotoHawk_lib/Calibration & Probing Blocks/motohawk_calibration  nam='VDO_Gauge_StartupDelay'  val=2  storage=Calibration  show_more=on  name_source=Use Parameter  data_type=double  read_level=1  write_level=1  ovr_cals=on  view_as=Number  enum_struct={'Disabled', 'Enabled'}  vector_style=Wide Row  use_help_units=off  help=''  units=''  use_header_enum=off  row_header_enum={}  col_header_enum={}  use_min_max=off  min_val=0  max_val=7  use_precision=off  precision=''  gain=1  offset=0  exp=1  use_mototune_group=on  mototune_group='Gauges'
  motohawk_calibration2 : MotoHawk_lib/Calibration & Probing Blocks/motohawk_calibration  nam='VDO_Gauge_Brightness'  val=5  storage=Calibration  show_more=on  name_source=Use Parameter  data_type=uint16  read_level=1  write_level=1  ovr_cals=on  view_as=Number  enum_struct={'Disabled', 'Enabled'}  vector_style=Wide Row  use_help_units=off  help=''  units=''  use_header_enum=off  row_header_enum={}  col_header_enum={}  use_min_max=on  min_val=0  max_val=7  use_precision=off  precision=''  gain=1  offset=0  exp=1  use_mototune_group=on  mototune_group='Gauges'
  motohawk_fault_action : MotoHawk_lib/Fault Management Blocks/motohawk_fault_action  nam='Battery_Warning'  output_status=on  eval_nam=Battery_Warning
  motohawk_fault_action1 : MotoHawk_lib/Fault Management Blocks/motohawk_fault_action  nam='Bat_limit_high'  output_status=on  eval_nam=Bat_limit_high
  motohawk_fault_action2 : MotoHawk_lib/Fault Management Blocks/motohawk_fault_action  nam='Bat_limit_low'  output_status=on  eval_nam=Bat_limit_low
  motohawk_fault_status : MotoHawk_lib/Fault Management Blocks/motohawk_fault_status  source=Lookup By Name  nam='GroundFault'  status=Active
  motohawk_fault_status1 : MotoHawk_lib/Fault Management Blocks/motohawk_fault_status  source=Lookup By Name  nam='Battery_UnderTemp'  status=Active
  motohawk_fault_status2 : MotoHawk_lib/Fault Management Blocks/motohawk_fault_status  source=Lookup By Name  nam='Battery_OverTemp'  status=Active
  motohawk_fault_status3 : MotoHawk_lib/Fault Management Blocks/motohawk_fault_status  source=Lookup By Name  nam='Inverter_OverTemp'  status=Active
  motohawk_fault_statuses : MotoHawk_lib/Fault Management Blocks/motohawk_fault_statuses  nam=motohawk_get_faults(bdroot)  status=Active
  tag scope: TimeSinceKeyOn=global
  wires:
  Inputs/1 -> Bus Selector/1
  Bus Selector/1 -> Gain/1  "<VehicleSpeed>"
  Gain/1 -> Saturation/1
  Saturation/1 -> Abs/1
  Data Type Conversion/1 -> VDO Gauge Write/1
  Bus Selector/2 -> Gain1/1, [SOC]  "<SOC>"
  Gain1/1 -> Saturation1/1
  Saturation1/1 -> Data Type Conversion1/1
  Data Type Conversion1/1 -> VDO Gauge Write2/1
  Bus Selector/3 -> Gain2/1  "<LVVoltage>"
  Gain2/1 -> Saturation2/1
  Saturation2/1 -> Data Type Conversion2/1
  Data Type Conversion2/1 -> VDO Gauge Write1/1
  motohawk_fault_statuses/1 -> Logical Operator1/1
  Logical Operator1/1 -> Data Type Conversion4/1
  Abs/1 -> Data Type Conversion/1
  Bus Selector/4 -> [TimeSinceKeyOn]  "<TimeSinceKeyOn>"
  [TimeSinceKeyOn] -> Relational Operator/2
  Relational Operator/1 -> Switch1/2
  Constant6/1 -> Switch1/3
  Switch1/1 -> Data Type Conversion5/1
  Bus Selector/5 -> Logical Operator2/1, Product/2  "<ContactorStatus>"
  Bus Selector/6 -> Logical Operator3/1  "<DriveReady>"
  Constant2/1 -> VDO Gauge LED Alarm Write/3  "Engine Warning"
  Data Type Conversion4/1 -> VDO Gauge LED Alarm Write/4  "Data"
  Data Type Conversion3/1 -> VDO Gauge LED Alarm Write/6  "Volt"
  Logical Operator3/1 -> Data Type Conversion7/1
  Constant3/1 -> VDO Gauge LED Alarm Write/1
  Data Type Conversion7/1 -> VDO Gauge LED Alarm Write/2
  motohawk_calibration1/1 -> Relational Operator/1
  Data Type Conversion8/1 -> VDO Gauge LED Alarm Write/5
  Product/1 -> Data Type Conversion8/1
  Add2/1 -> Saturation3/1  "Fuel"
  motohawk_calibration2/1 -> Switch1/1
  motohawk_fault_status/1 -> Switch2/2
  Logical Operator2/1 -> Switch2/3
  Switch2/1 -> Data Type Conversion3/1
  Constant4/1 -> Switch2/1
  Data Type Conversion5/1 -> VDO Gauge Brightness/1
  motohawk_fault_status1/1 -> Logical Operator4/1
  motohawk_fault_status2/1 -> Logical Operator4/2
  Logical Operator4/1 -> Switch3/2
  Constant7/1 -> Switch3/1
  Constant8/1 -> Switch3/3
  motohawk_fault_status3/1 -> Data Type Conversion9/1  "Temperature"
  Switch3/1 -> Data Type Conversion6/1
  MinMax/1 -> VDO Gauge LED Alarm Write/7
  Data Type Conversion9/1 -> MinMax/1
  Data Type Conversion6/1 -> MinMax/2
  Data Type Conversion10/1 -> VDO Gauge LED Alarm Write/8
  motohawk_fault_action/1 -> Add2/1
  Saturation3/1 -> Product/1
  motohawk_fault_action2/1 -> Add2/2
  motohawk_fault_action1/1 -> Add2/3
  Outputs/1 -> Bus Selector1/1
  Bus Selector1/1 -> Data Type Conversion10/1  "<InReverse>"
